simulink model "WhirlyBird"  (R2016a)
settings: Solver=VariableStepAuto  StartTime=0.0  StopTime=10000  RelTol=1e-3
undefined symbols (not defined in the file or in its folder): drawWhirly
libraries: simulink x3
settings Model: Creator=Jacob  LastModifiedBy=Jacob

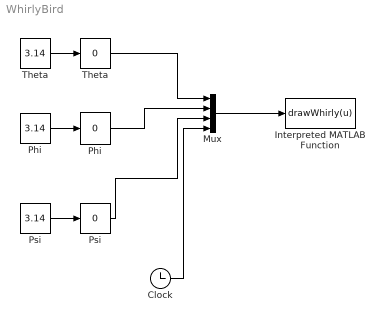
== system WhirlyBird ==
  Clock : Clock
  Interpreted MATLAB Function : MATLABFcn  MATLABFcn=drawWhirly(u)  OutputDimensions=0
  Mux : Mux
  Phi : Constant  Value=3.14  SampleTime=1
  "Phi " : simulink/Math Operations/Slider Gain  low=0  gain=0  high=2
  Psi : Constant  Value=3.14  SampleTime=1
  "Psi " : simulink/Math Operations/Slider Gain  low=0  gain=0  high=2
  Theta : Constant  Value=3.14  SampleTime=1
  "Theta " : simulink/Math Operations/Slider Gain  low=0  gain=0  high=2
  wires:
  Mux/1 -> Interpreted MATLAB Function/1
  Clock/1 -> Mux/4
  Psi/1 -> "Psi "/1
  "Psi "/1 -> Mux/3
  Theta/1 -> "Theta "/1
  "Phi "/1 -> Mux/2
  "Theta "/1 -> Mux/1
  Phi/1 -> "Phi "/1
